simulink model "pd_controller_j2n6s300"  (R2015a)
settings: Solver=ode45  StartTime=0.0  StopTime=0.3  RelTol=1e-3
undefined symbols (not defined in the file or in its folder): eom
libraries: simulink x6
settings Model: Creator=user  LastModifiedBy=user

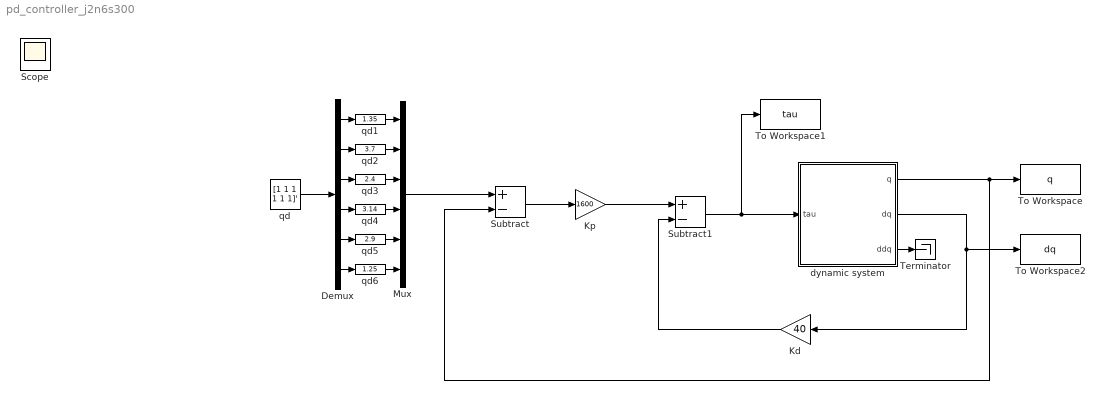
== system pd_controller_j2n6s300 ==
  Demux : Demux  Outputs=6
  Kd : Gain  Gain=40
  Kp : Gain  Gain=1600
  Mux : Mux  Inputs=6
  Subtract : Sum  Inputs=+-
  Subtract1 : Sum  Inputs=+-
  Terminator : Terminator
  To Workspace : ToWorkspace  VariableName=q  SaveFormat=Timeseries  SampleTime=-1
  To Workspace1 : ToWorkspace  VariableName=tau  SaveFormat=Timeseries  SampleTime=-1
  To Workspace2 : ToWorkspace  VariableName=dq  SaveFormat=Timeseries  SampleTime=-1
  dynamic system : Subsystem  mask{Ts=0.01, phi0=[0.0 2.9 1.3 4.2 1.4 0.0]', dphi0=[0 0 0 0 0 0]'}
      mask prompts: Ts "Sample time"; phi0 "Initial joint positions"; dphi0 "Initial joint velocities"
  qd : Constant  Value=[1 1 1 1 1 1]'
  qd1 : simulink/Math Operations/Slider Gain  low=-2  gain=1.35  high=3.14
  qd2 : simulink/Math Operations/Slider Gain  low=-2  gain=3.7  high=3.7
  qd3 : simulink/Math Operations/Slider Gain  low=-2  gain=2.4  high=2.4
  qd4 : simulink/Math Operations/Slider Gain  low=-2  gain=3.14  high=3.14
  qd5 : simulink/Math Operations/Slider Gain  low=-2  gain=2.9  high=2.9
  qd6 : simulink/Math Operations/Slider Gain  low=-3.14  gain=1.25  high=2
  Scope : Scope
  wires:
  dynamic system/1(q) -> Subtract/2, To Workspace/1
  dynamic system/3(ddq) -> Terminator/1
  Demux/2 -> qd2/1
  Demux/4 -> qd4/1
  Demux/6 -> qd6/1
  qd6/1 -> Mux/6
  qd5/1 -> Mux/5
  qd4/1 -> Mux/4
  qd3/1 -> Mux/3
  qd2/1 -> Mux/2
  qd1/1 -> Mux/1
  qd/1 -> Demux/1
  Mux/1 -> Subtract/1
  Demux/3 -> qd3/1
  Demux/5 -> qd5/1
  Subtract1/1 -> dynamic system/1(tau), To Workspace1/1
  Demux/1 -> qd1/1
  dynamic system/2(dq) -> To Workspace2/1, Kd/1
  Kp/1 -> Subtract1/1
  Subtract/1 -> Kp/1
  Kd/1 -> Subtract1/2

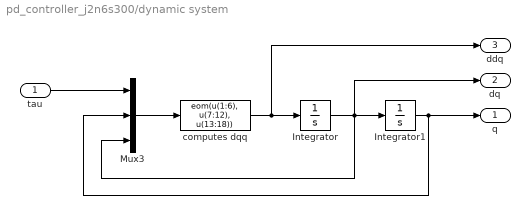
== system pd_controller_j2n6s300/dynamic system ==
  tau : Inport
  Integrator : Integrator  InitialCondition=dphi0
  Integrator1 : Integrator  InitialCondition=phi0
  Mux3 : Mux  Inputs=3
  computes dqq : MATLABFcn  MATLABFcn=eom(u(1:6), u(7:12), u(13:18))  OutputDimensions=[6,1]  Output1D=off
  q : Outport
  dq : Outport  Port=2
  ddq : Outport  Port=3
  wires:
  Integrator/1 -> Mux3/3, dq/1, Integrator1/1
  tau/1 -> Mux3/1
  Integrator1/1 -> Mux3/2, q/1
  Mux3/1 -> computes dqq/1
  computes dqq/1 -> ddq/1, Integrator/1
